simulink model "TST_APP_PlausBrk"  (R2016b)
settings: Solver=FixedStepDiscrete  StartTime=0.0  StopTime=simTime  FixedStep=sampleTime  RelTol=1e-3
values from neighbouring files (symbols this model uses):
  testCase = 1    [initTST_APP_PlausBrk_001.m]    (also in initTST_APP_PlausBrk_002.m = 2; initTST_APP_PlausBrk_003.m = 3; initTST_APP_PlausBrk_004.m = 4; initTST_APP_PlausBrk_005.m = 5)
libraries: simulink x25, UnitTest_Lib x18
(part 1 of 2)
settings Model: Creator=liangyunbo  LastModifiedBy=liangyunbo
settings DebuggingCC: SignalRangeChecking=error

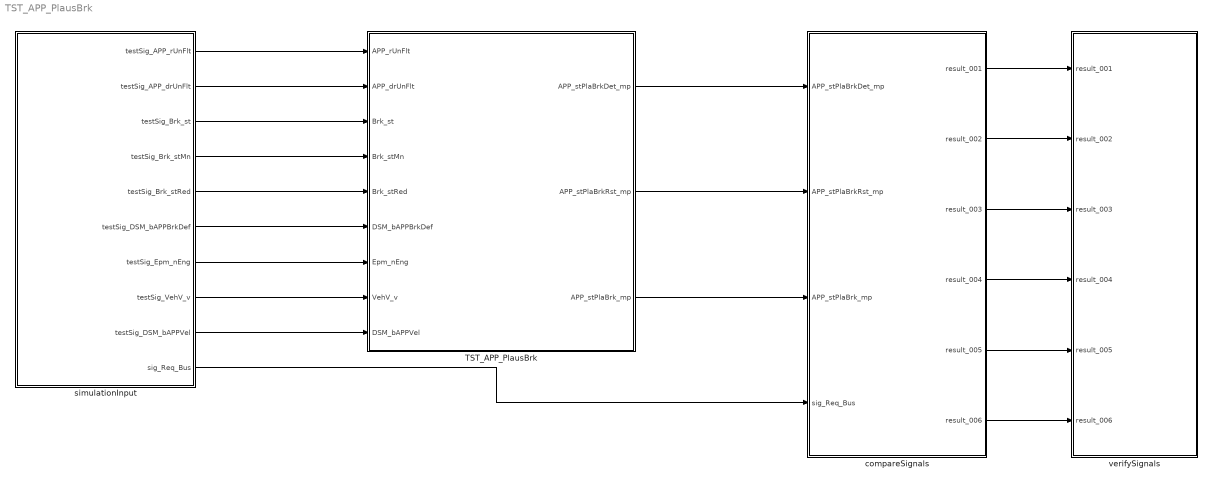
== system TST_APP_PlausBrk ==
  TST_APP_PlausBrk : Subsystem
  compareSignals : Subsystem
  simulationInput : Subsystem
  verifySignals : Subsystem
  wires:
  simulationInput/1(testSig_APP_rUnFlt) -> TST_APP_PlausBrk/1(APP_rUnFlt)
  simulationInput/2(testSig_APP_drUnFlt) -> TST_APP_PlausBrk/2(APP_drUnFlt)
  simulationInput/3(testSig_Brk_st) -> TST_APP_PlausBrk/3(Brk_st)
  simulationInput/4(testSig_Brk_stMn) -> TST_APP_PlausBrk/4(Brk_stMn)
  simulationInput/5(testSig_Brk_stRed) -> TST_APP_PlausBrk/5(Brk_stRed)
  simulationInput/6(testSig_DSM_bAPPBrkDef) -> TST_APP_PlausBrk/6(DSM_bAPPBrkDef)
  simulationInput/7(testSig_Epm_nEng) -> TST_APP_PlausBrk/7(Epm_nEng)
  simulationInput/8(testSig_VehV_v) -> TST_APP_PlausBrk/8(VehV_v)
  simulationInput/9(testSig_DSM_bAPPVel) -> TST_APP_PlausBrk/9(DSM_bAPPVel)
  TST_APP_PlausBrk/1(APP_stPlaBrkDet_mp) -> compareSignals/1(APP_stPlaBrkDet_mp)
  TST_APP_PlausBrk/2(APP_stPlaBrkRst_mp) -> compareSignals/2(APP_stPlaBrkRst_mp)
  TST_APP_PlausBrk/3(APP_stPlaBrk_mp) -> compareSignals/3(APP_stPlaBrk_mp)
  simulationInput/10(sig_Req_Bus) -> compareSignals/4(sig_Req_Bus)
  compareSignals/1(result_001) -> verifySignals/1(result_001)
  compareSignals/2(result_002) -> verifySignals/2(result_002)
  compareSignals/3(result_003) -> verifySignals/3(result_003)
  compareSignals/4(result_004) -> verifySignals/4(result_004)
  compareSignals/5(result_005) -> verifySignals/5(result_005)
  compareSignals/6(result_006) -> verifySignals/6(result_006)

== system TST_APP_PlausBrk/TST_APP_PlausBrk ==
  APP_rUnFlt : Inport
  APP_drUnFlt : Inport  Port=2
  Brk_st : Inport  Port=3
  Brk_stMn : Inport  Port=4
  Brk_stRed : Inport  Port=5
  DSM_bAPPBrkDef : Inport  Port=6
  Epm_nEng : Inport  Port=7
  VehV_v : Inport  Port=8
  DSM_bAPPVel : Inport  Port=9
  APP_PlausBrk : ModelReference  ModelNameDialog=APP_PlausBrk  SimulationMode=Normal  ModelReferenceVersion=1.27  TriggerPortName=function  TriggerPortTriggerType=function-call  TriggerPortStatesWhenEnabling=held
  Function_Call : simulink/Ports & Subsystems/Function-Call Generator  sample_time=sampleTime  numberOfIterations=1
  APP_stPlaBrkDet_mp : Outport
  APP_stPlaBrkRst_mp : Outport  Port=2
  APP_stPlaBrk_mp : Outport  Port=3
  wires:
  Function_Call/1 -> APP_PlausBrk/Trigger
  APP_rUnFlt/1 -> APP_PlausBrk/1
  APP_drUnFlt/1 -> APP_PlausBrk/2
  Brk_st/1 -> APP_PlausBrk/3
  Brk_stMn/1 -> APP_PlausBrk/4
  Brk_stRed/1 -> APP_PlausBrk/5
  DSM_bAPPBrkDef/1 -> APP_PlausBrk/6
  Epm_nEng/1 -> APP_PlausBrk/7
  VehV_v/1 -> APP_PlausBrk/8
  DSM_bAPPVel/1 -> APP_PlausBrk/9
  APP_PlausBrk/1 -> APP_stPlaBrkDet_mp/1
  APP_PlausBrk/2 -> APP_stPlaBrkRst_mp/1
  APP_PlausBrk/3 -> APP_stPlaBrk_mp/1

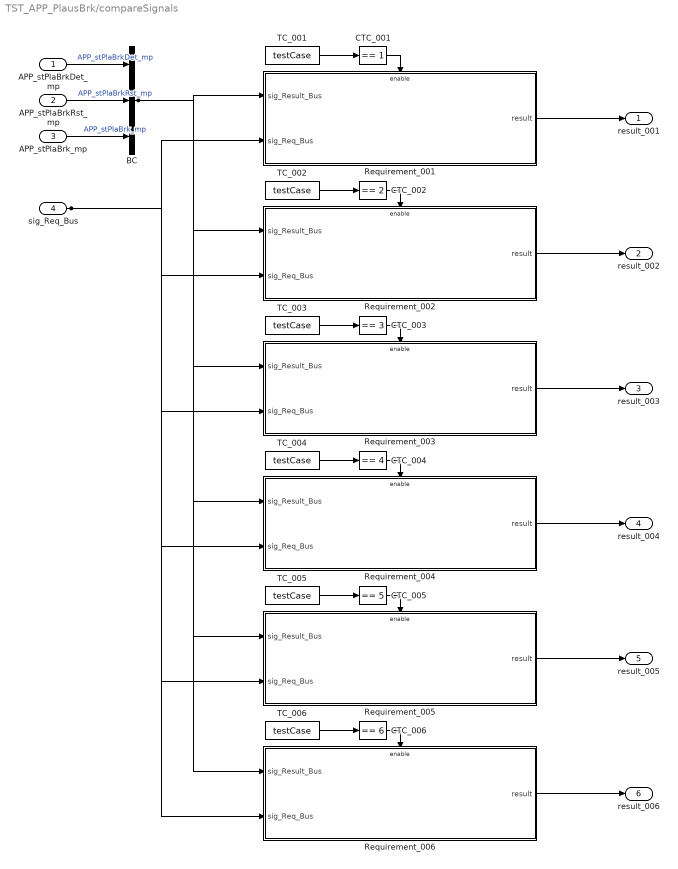
== system TST_APP_PlausBrk/compareSignals ==
  APP_stPlaBrkDet_mp : Inport
  APP_stPlaBrkRst_mp : Inport  Port=2
  APP_stPlaBrk_mp : Inport  Port=3
  sig_Req_Bus : Inport  Port=4
  BC : BusCreator  Inputs=3
  CTC_001 : simulink/Logic and Bit Operations/Compare To Constant  relop===  const=1  OutDataTypeStr=boolean
  CTC_002 : simulink/Logic and Bit Operations/Compare To Constant  relop===  const=2  OutDataTypeStr=boolean
  CTC_003 : simulink/Logic and Bit Operations/Compare To Constant  relop===  const=3  OutDataTypeStr=boolean
  CTC_004 : simulink/Logic and Bit Operations/Compare To Constant  relop===  const=4  OutDataTypeStr=boolean
  CTC_005 : simulink/Logic and Bit Operations/Compare To Constant  relop===  const=5  OutDataTypeStr=boolean
  CTC_006 : simulink/Logic and Bit Operations/Compare To Constant  relop===  const=6  OutDataTypeStr=boolean
  Requirement_001 : Subsystem
  Requirement_002 : Subsystem
  Requirement_003 : Subsystem
  Requirement_004 : Subsystem
  Requirement_005 : Subsystem
  Requirement_006 : Subsystem
  TC_001 : Constant  Value=testCase
  TC_002 : Constant  Value=testCase
  TC_003 : Constant  Value=testCase
  TC_004 : Constant  Value=testCase
  TC_005 : Constant  Value=testCase
  TC_006 : Constant  Value=testCase
  result_001 : Outport
  result_002 : Outport  Port=2
  result_003 : Outport  Port=3
  result_004 : Outport  Port=4
  result_005 : Outport  Port=5
  result_006 : Outport  Port=6
  wires:
  APP_stPlaBrkDet_mp/1 -> BC/1  "APP_stPlaBrkDet_mp"
  APP_stPlaBrkRst_mp/1 -> BC/2  "APP_stPlaBrkRst_mp"
  APP_stPlaBrk_mp/1 -> BC/3  "APP_stPlaBrk_mp"
  TC_001/1 -> CTC_001/1
  CTC_001/1 -> Requirement_001/Enable
  sig_Req_Bus/1 -> Requirement_001/2(sig_Req_Bus), Requirement_002/2(sig_Req_Bus), Requirement_003/2(sig_Req_Bus), Requirement_004/2(sig_Req_Bus), Requirement_005/2(sig_Req_Bus), Requirement_006/2(sig_Req_Bus)
  BC/1 -> Requirement_001/1(sig_Result_Bus), Requirement_002/1(sig_Result_Bus), Requirement_003/1(sig_Result_Bus), Requirement_004/1(sig_Result_Bus), Requirement_005/1(sig_Result_Bus), Requirement_006/1(sig_Result_Bus)
  Requirement_001/1(result) -> result_001/1
  TC_002/1 -> CTC_002/1
  CTC_002/1 -> Requirement_002/Enable
  Requirement_002/1(result) -> result_002/1
  TC_003/1 -> CTC_003/1
  CTC_003/1 -> Requirement_003/Enable
  Requirement_003/1(result) -> result_003/1
  TC_004/1 -> CTC_004/1
  CTC_004/1 -> Requirement_004/Enable
  Requirement_004/1(result) -> result_004/1
  TC_005/1 -> CTC_005/1
  CTC_005/1 -> Requirement_005/Enable
  Requirement_005/1(result) -> result_005/1
  TC_006/1 -> CTC_006/1
  CTC_006/1 -> Requirement_006/Enable
  Requirement_006/1(result) -> result_006/1

== system TST_APP_PlausBrk/simulationInput ==
  BS : BusSelector  OutputSignals=testSig_APP_rUnFlt,testSig_APP_drUnFlt,testSig_Brk_st,testSig_Brk_stMn,testSig_Brk_stRed,testSig_DSM_bAPPBrkDef,testSig_Epm_nEng,testSig_VehV_v,testSig_DSM_bAPPVel
  MPSw : MultiPortSwitch  Inputs=6  SaturateOnIntegerOverflow=on  InputSameDT=on
  TestCase : Constant  Value=testCase
  testSignals_R001 : Subsystem
  testSignals_R002 : Subsystem
  testSignals_R003 : Subsystem
  testSignals_R004 : Subsystem
  testSignals_R005 : Subsystem
  testSignals_R006 : Subsystem
  testSig_APP_rUnFlt : Outport
  testSig_APP_drUnFlt : Outport  Port=2
  testSig_Brk_st : Outport  Port=3
  testSig_Brk_stMn : Outport  Port=4
  testSig_Brk_stRed : Outport  Port=5
  testSig_DSM_bAPPBrkDef : Outport  Port=6
  testSig_Epm_nEng : Outport  Port=7
  testSig_VehV_v : Outport  Port=8
  testSig_DSM_bAPPVel : Outport  Port=9
  sig_Req_Bus : Outport  Port=10
  wires:
  BS/1 -> testSig_APP_rUnFlt/1  "<testSig_APP_rUnFlt>"
  BS/2 -> testSig_APP_drUnFlt/1  "<testSig_APP_drUnFlt>"
  BS/3 -> testSig_Brk_st/1  "<testSig_Brk_st>"
  BS/4 -> testSig_Brk_stMn/1  "<testSig_Brk_stMn>"
  BS/5 -> testSig_Brk_stRed/1  "<testSig_Brk_stRed>"
  BS/6 -> testSig_DSM_bAPPBrkDef/1  "<testSig_DSM_bAPPBrkDef>"
  BS/7 -> testSig_Epm_nEng/1  "<testSig_Epm_nEng>"
  BS/8 -> testSig_VehV_v/1  "<testSig_VehV_v>"
  BS/9 -> testSig_DSM_bAPPVel/1  "<testSig_DSM_bAPPVel>"
  MPSw/1 -> BS/1, sig_Req_Bus/1
  TestCase/1 -> MPSw/1
  testSignals_R001/1(testSignals) -> MPSw/2
  testSignals_R002/1(testSignals) -> MPSw/3
  testSignals_R003/1(testSignals) -> MPSw/4
  testSignals_R004/1(testSignals) -> MPSw/5
  testSignals_R005/1(testSignals) -> MPSw/6
  testSignals_R006/1(testSignals) -> MPSw/7

== system TST_APP_PlausBrk/verifySignals ==
  result_001 : Inport
  result_002 : Inport  Port=2
  result_003 : Inport  Port=3
  result_004 : Inport  Port=4
  result_005 : Inport  Port=5
  result_006 : Inport  Port=6
  Assertion_001 : Assertion  Enabled=off
  Assertion_002 : Assertion  Enabled=off
  Assertion_003 : Assertion  Enabled=off
  Assertion_004 : Assertion  Enabled=off
  Assertion_005 : Assertion  Enabled=off
  Assertion_006 : Assertion  Enabled=off
  wires:
  result_001/1 -> Assertion_001/1
  result_002/1 -> Assertion_002/1
  result_003/1 -> Assertion_003/1
  result_004/1 -> Assertion_004/1
  result_005/1 -> Assertion_005/1
  result_006/1 -> Assertion_006/1

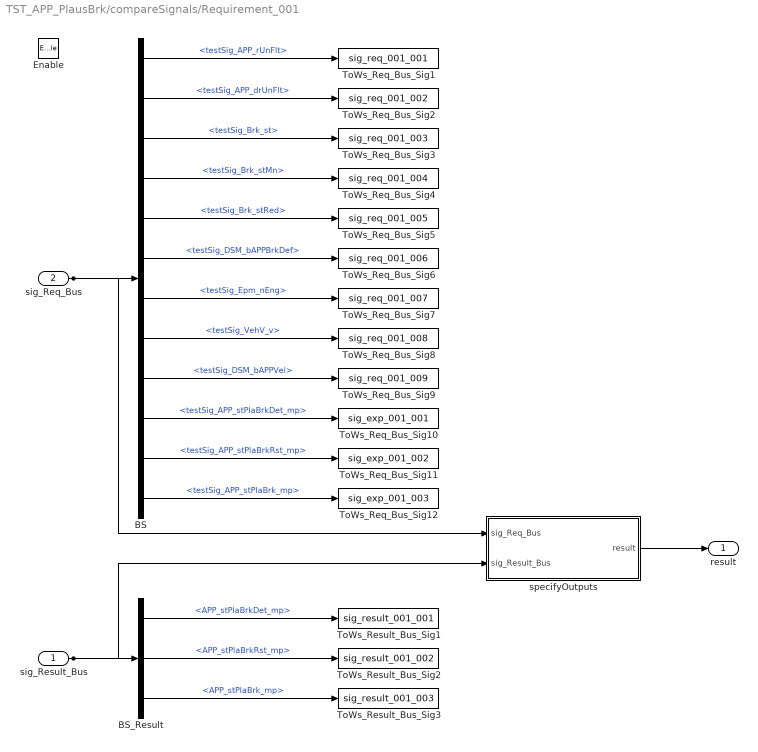
== system TST_APP_PlausBrk/compareSignals/Requirement_001 ==
  sig_Result_Bus : Inport
  sig_Req_Bus : Inport  Port=2
  Enable : EnablePort
  BS : BusSelector  OutputSignals=testSig_APP_rUnFlt,testSig_APP_drUnFlt,testSig_Brk_st,testSig_Brk_stMn,testSig_Brk_stRed,testSig_DSM_bAPPBrkDef,testSig_Epm_nEng,testSig_VehV_v,testSig_DSM_bAPPVel,testSig_APP_stPlaBrkDet_mp,testSig_APP_stPlaBrkRst_mp,testSig_APP_stPlaBrk_mp
  BS_Result : BusSelector  OutputSignals=APP_stPlaBrkDet_mp,APP_stPlaBrkRst_mp,APP_stPlaBrk_mp
  ToWs_Req_Bus_Sig1 : ToWorkspace  VariableName=sig_req_001_001  SaveFormat=Structure With Time
  ToWs_Req_Bus_Sig10 : ToWorkspace  VariableName=sig_exp_001_001  SaveFormat=Structure With Time
  ToWs_Req_Bus_Sig11 : ToWorkspace  VariableName=sig_exp_001_002  SaveFormat=Structure With Time
  ToWs_Req_Bus_Sig12 : ToWorkspace  VariableName=sig_exp_001_003  SaveFormat=Structure With Time
  ToWs_Req_Bus_Sig2 : ToWorkspace  VariableName=sig_req_001_002  SaveFormat=Structure With Time
  ToWs_Req_Bus_Sig3 : ToWorkspace  VariableName=sig_req_001_003  SaveFormat=Structure With Time
  ToWs_Req_Bus_Sig4 : ToWorkspace  VariableName=sig_req_001_004  SaveFormat=Structure With Time
  ToWs_Req_Bus_Sig5 : ToWorkspace  VariableName=sig_req_001_005  SaveFormat=Structure With Time
  ToWs_Req_Bus_Sig6 : ToWorkspace  VariableName=sig_req_001_006  SaveFormat=Structure With Time
  ToWs_Req_Bus_Sig7 : ToWorkspace  VariableName=sig_req_001_007  SaveFormat=Structure With Time
  ToWs_Req_Bus_Sig8 : ToWorkspace  VariableName=sig_req_001_008  SaveFormat=Structure With Time
  ToWs_Req_Bus_Sig9 : ToWorkspace  VariableName=sig_req_001_009  SaveFormat=Structure With Time
  ToWs_Result_Bus_Sig1 : ToWorkspace  VariableName=sig_result_001_001  SaveFormat=Structure With Time
  ToWs_Result_Bus_Sig2 : ToWorkspace  VariableName=sig_result_001_002  SaveFormat=Structure With Time
  ToWs_Result_Bus_Sig3 : ToWorkspace  VariableName=sig_result_001_003  SaveFormat=Structure With Time
  specifyOutputs : Subsystem
  result : Outport
  wires:
  sig_Req_Bus/1 -> BS/1, specifyOutputs/1(sig_Req_Bus)
  BS/1 -> ToWs_Req_Bus_Sig1/1  "<testSig_APP_rUnFlt>"
  BS/2 -> ToWs_Req_Bus_Sig2/1  "<testSig_APP_drUnFlt>"
  BS/3 -> ToWs_Req_Bus_Sig3/1  "<testSig_Brk_st>"
  BS/4 -> ToWs_Req_Bus_Sig4/1  "<testSig_Brk_stMn>"
  BS/5 -> ToWs_Req_Bus_Sig5/1  "<testSig_Brk_stRed>"
  BS/6 -> ToWs_Req_Bus_Sig6/1  "<testSig_DSM_bAPPBrkDef>"
  BS/7 -> ToWs_Req_Bus_Sig7/1  "<testSig_Epm_nEng>"
  BS/8 -> ToWs_Req_Bus_Sig8/1  "<testSig_VehV_v>"
  BS/9 -> ToWs_Req_Bus_Sig9/1  "<testSig_DSM_bAPPVel>"
  BS/10 -> ToWs_Req_Bus_Sig10/1  "<testSig_APP_stPlaBrkDet_mp>"
  BS/11 -> ToWs_Req_Bus_Sig11/1  "<testSig_APP_stPlaBrkRst_mp>"
  BS/12 -> ToWs_Req_Bus_Sig12/1  "<testSig_APP_stPlaBrk_mp>"
  sig_Result_Bus/1 -> BS_Result/1, specifyOutputs/2(sig_Result_Bus)
  BS_Result/1 -> ToWs_Result_Bus_Sig1/1  "<APP_stPlaBrkDet_mp>"
  BS_Result/2 -> ToWs_Result_Bus_Sig2/1  "<APP_stPlaBrkRst_mp>"
  BS_Result/3 -> ToWs_Result_Bus_Sig3/1  "<APP_stPlaBrk_mp>"
  specifyOutputs/1(result) -> result/1

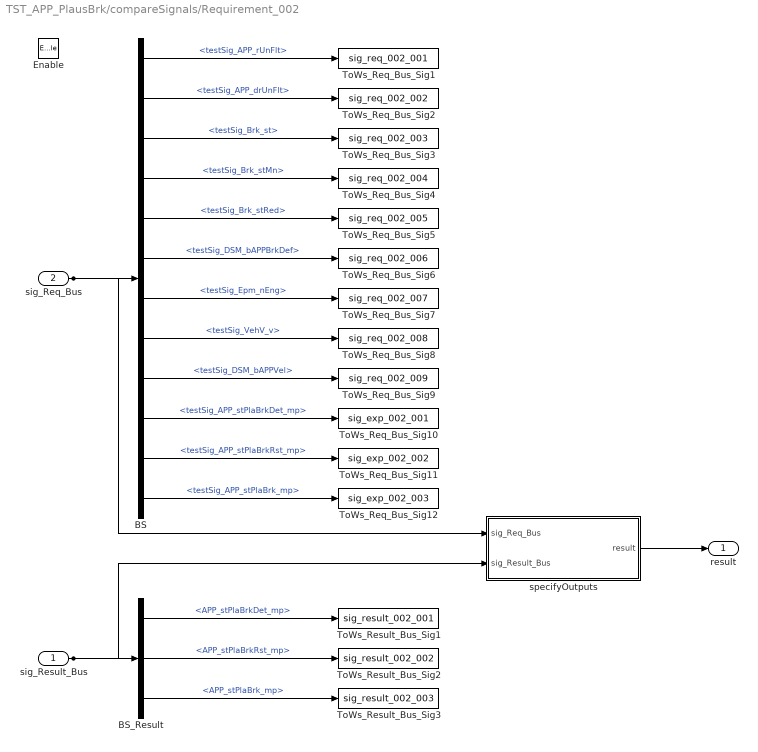
== system TST_APP_PlausBrk/compareSignals/Requirement_002 ==
  sig_Result_Bus : Inport
  sig_Req_Bus : Inport  Port=2
  Enable : EnablePort
  BS : BusSelector  OutputSignals=testSig_APP_rUnFlt,testSig_APP_drUnFlt,testSig_Brk_st,testSig_Brk_stMn,testSig_Brk_stRed,testSig_DSM_bAPPBrkDef,testSig_Epm_nEng,testSig_VehV_v,testSig_DSM_bAPPVel,testSig_APP_stPlaBrkDet_mp,testSig_APP_stPlaBrkRst_mp,testSig_APP_stPlaBrk_mp
  BS_Result : BusSelector  OutputSignals=APP_stPlaBrkDet_mp,APP_stPlaBrkRst_mp,APP_stPlaBrk_mp
  ToWs_Req_Bus_Sig1 : ToWorkspace  VariableName=sig_req_002_001  SaveFormat=Structure With Time
  ToWs_Req_Bus_Sig10 : ToWorkspace  VariableName=sig_exp_002_001  SaveFormat=Structure With Time
  ToWs_Req_Bus_Sig11 : ToWorkspace  VariableName=sig_exp_002_002  SaveFormat=Structure With Time
  ToWs_Req_Bus_Sig12 : ToWorkspace  VariableName=sig_exp_002_003  SaveFormat=Structure With Time
  ToWs_Req_Bus_Sig2 : ToWorkspace  VariableName=sig_req_002_002  SaveFormat=Structure With Time
  ToWs_Req_Bus_Sig3 : ToWorkspace  VariableName=sig_req_002_003  SaveFormat=Structure With Time
  ToWs_Req_Bus_Sig4 : ToWorkspace  VariableName=sig_req_002_004  SaveFormat=Structure With Time
  ToWs_Req_Bus_Sig5 : ToWorkspace  VariableName=sig_req_002_005  SaveFormat=Structure With Time
  ToWs_Req_Bus_Sig6 : ToWorkspace  VariableName=sig_req_002_006  SaveFormat=Structure With Time
  ToWs_Req_Bus_Sig7 : ToWorkspace  VariableName=sig_req_002_007  SaveFormat=Structure With Time
  ToWs_Req_Bus_Sig8 : ToWorkspace  VariableName=sig_req_002_008  SaveFormat=Structure With Time
  ToWs_Req_Bus_Sig9 : ToWorkspace  VariableName=sig_req_002_009  SaveFormat=Structure With Time
  ToWs_Result_Bus_Sig1 : ToWorkspace  VariableName=sig_result_002_001  SaveFormat=Structure With Time
  ToWs_Result_Bus_Sig2 : ToWorkspace  VariableName=sig_result_002_002  SaveFormat=Structure With Time
  ToWs_Result_Bus_Sig3 : ToWorkspace  VariableName=sig_result_002_003  SaveFormat=Structure With Time
  specifyOutputs : Subsystem
  result : Outport
  wires:
  sig_Req_Bus/1 -> BS/1, specifyOutputs/1(sig_Req_Bus)
  BS/1 -> ToWs_Req_Bus_Sig1/1  "<testSig_APP_rUnFlt>"
  BS/2 -> ToWs_Req_Bus_Sig2/1  "<testSig_APP_drUnFlt>"
  BS/3 -> ToWs_Req_Bus_Sig3/1  "<testSig_Brk_st>"
  BS/4 -> ToWs_Req_Bus_Sig4/1  "<testSig_Brk_stMn>"
  BS/5 -> ToWs_Req_Bus_Sig5/1  "<testSig_Brk_stRed>"
  BS/6 -> ToWs_Req_Bus_Sig6/1  "<testSig_DSM_bAPPBrkDef>"
  BS/7 -> ToWs_Req_Bus_Sig7/1  "<testSig_Epm_nEng>"
  BS/8 -> ToWs_Req_Bus_Sig8/1  "<testSig_VehV_v>"
  BS/9 -> ToWs_Req_Bus_Sig9/1  "<testSig_DSM_bAPPVel>"
  BS/10 -> ToWs_Req_Bus_Sig10/1  "<testSig_APP_stPlaBrkDet_mp>"
  BS/11 -> ToWs_Req_Bus_Sig11/1  "<testSig_APP_stPlaBrkRst_mp>"
  BS/12 -> ToWs_Req_Bus_Sig12/1  "<testSig_APP_stPlaBrk_mp>"
  sig_Result_Bus/1 -> BS_Result/1, specifyOutputs/2(sig_Result_Bus)
  BS_Result/1 -> ToWs_Result_Bus_Sig1/1  "<APP_stPlaBrkDet_mp>"
  BS_Result/2 -> ToWs_Result_Bus_Sig2/1  "<APP_stPlaBrkRst_mp>"
  BS_Result/3 -> ToWs_Result_Bus_Sig3/1  "<APP_stPlaBrk_mp>"
  specifyOutputs/1(result) -> result/1

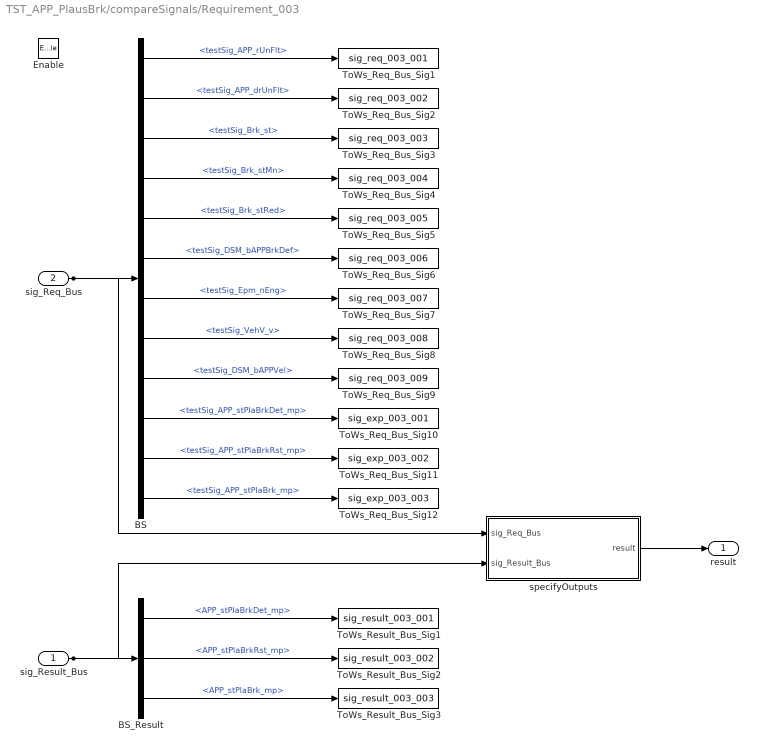
== system TST_APP_PlausBrk/compareSignals/Requirement_003 ==
  sig_Result_Bus : Inport
  sig_Req_Bus : Inport  Port=2
  Enable : EnablePort
  BS : BusSelector  OutputSignals=testSig_APP_rUnFlt,testSig_APP_drUnFlt,testSig_Brk_st,testSig_Brk_stMn,testSig_Brk_stRed,testSig_DSM_bAPPBrkDef,testSig_Epm_nEng,testSig_VehV_v,testSig_DSM_bAPPVel,testSig_APP_stPlaBrkDet_mp,testSig_APP_stPlaBrkRst_mp,testSig_APP_stPlaBrk_mp
  BS_Result : BusSelector  OutputSignals=APP_stPlaBrkDet_mp,APP_stPlaBrkRst_mp,APP_stPlaBrk_mp
  ToWs_Req_Bus_Sig1 : ToWorkspace  VariableName=sig_req_003_001  SaveFormat=Structure With Time
  ToWs_Req_Bus_Sig10 : ToWorkspace  VariableName=sig_exp_003_001  SaveFormat=Structure With Time
  ToWs_Req_Bus_Sig11 : ToWorkspace  VariableName=sig_exp_003_002  SaveFormat=Structure With Time
  ToWs_Req_Bus_Sig12 : ToWorkspace  VariableName=sig_exp_003_003  SaveFormat=Structure With Time
  ToWs_Req_Bus_Sig2 : ToWorkspace  VariableName=sig_req_003_002  SaveFormat=Structure With Time
  ToWs_Req_Bus_Sig3 : ToWorkspace  VariableName=sig_req_003_003  SaveFormat=Structure With Time
  ToWs_Req_Bus_Sig4 : ToWorkspace  VariableName=sig_req_003_004  SaveFormat=Structure With Time
  ToWs_Req_Bus_Sig5 : ToWorkspace  VariableName=sig_req_003_005  SaveFormat=Structure With Time
  ToWs_Req_Bus_Sig6 : ToWorkspace  VariableName=sig_req_003_006  SaveFormat=Structure With Time
  ToWs_Req_Bus_Sig7 : ToWorkspace  VariableName=sig_req_003_007  SaveFormat=Structure With Time
  ToWs_Req_Bus_Sig8 : ToWorkspace  VariableName=sig_req_003_008  SaveFormat=Structure With Time
  ToWs_Req_Bus_Sig9 : ToWorkspace  VariableName=sig_req_003_009  SaveFormat=Structure With Time
  ToWs_Result_Bus_Sig1 : ToWorkspace  VariableName=sig_result_003_001  SaveFormat=Structure With Time
  ToWs_Result_Bus_Sig2 : ToWorkspace  VariableName=sig_result_003_002  SaveFormat=Structure With Time
  ToWs_Result_Bus_Sig3 : ToWorkspace  VariableName=sig_result_003_003  SaveFormat=Structure With Time
  specifyOutputs : Subsystem
  result : Outport
  wires:
  sig_Req_Bus/1 -> BS/1, specifyOutputs/1(sig_Req_Bus)
  BS/1 -> ToWs_Req_Bus_Sig1/1  "<testSig_APP_rUnFlt>"
  BS/2 -> ToWs_Req_Bus_Sig2/1  "<testSig_APP_drUnFlt>"
  BS/3 -> ToWs_Req_Bus_Sig3/1  "<testSig_Brk_st>"
  BS/4 -> ToWs_Req_Bus_Sig4/1  "<testSig_Brk_stMn>"
  BS/5 -> ToWs_Req_Bus_Sig5/1  "<testSig_Brk_stRed>"
  BS/6 -> ToWs_Req_Bus_Sig6/1  "<testSig_DSM_bAPPBrkDef>"
  BS/7 -> ToWs_Req_Bus_Sig7/1  "<testSig_Epm_nEng>"
  BS/8 -> ToWs_Req_Bus_Sig8/1  "<testSig_VehV_v>"
  BS/9 -> ToWs_Req_Bus_Sig9/1  "<testSig_DSM_bAPPVel>"
  BS/10 -> ToWs_Req_Bus_Sig10/1  "<testSig_APP_stPlaBrkDet_mp>"
  BS/11 -> ToWs_Req_Bus_Sig11/1  "<testSig_APP_stPlaBrkRst_mp>"
  BS/12 -> ToWs_Req_Bus_Sig12/1  "<testSig_APP_stPlaBrk_mp>"
  sig_Result_Bus/1 -> BS_Result/1, specifyOutputs/2(sig_Result_Bus)
  BS_Result/1 -> ToWs_Result_Bus_Sig1/1  "<APP_stPlaBrkDet_mp>"
  BS_Result/2 -> ToWs_Result_Bus_Sig2/1  "<APP_stPlaBrkRst_mp>"
  BS_Result/3 -> ToWs_Result_Bus_Sig3/1  "<APP_stPlaBrk_mp>"
  specifyOutputs/1(result) -> result/1

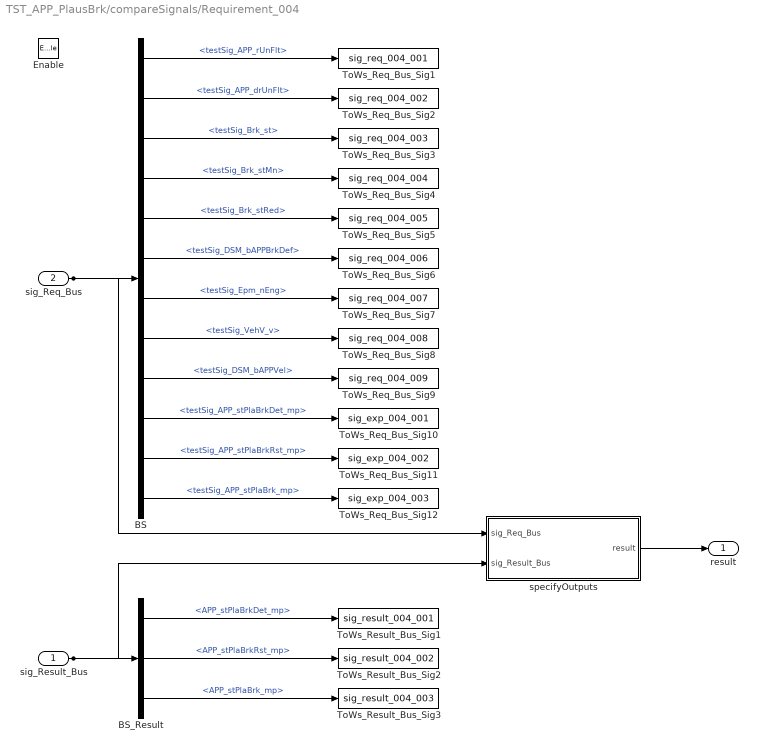
== system TST_APP_PlausBrk/compareSignals/Requirement_004 ==
  sig_Result_Bus : Inport
  sig_Req_Bus : Inport  Port=2
  Enable : EnablePort
  BS : BusSelector  OutputSignals=testSig_APP_rUnFlt,testSig_APP_drUnFlt,testSig_Brk_st,testSig_Brk_stMn,testSig_Brk_stRed,testSig_DSM_bAPPBrkDef,testSig_Epm_nEng,testSig_VehV_v,testSig_DSM_bAPPVel,testSig_APP_stPlaBrkDet_mp,testSig_APP_stPlaBrkRst_mp,testSig_APP_stPlaBrk_mp
  BS_Result : BusSelector  OutputSignals=APP_stPlaBrkDet_mp,APP_stPlaBrkRst_mp,APP_stPlaBrk_mp
  ToWs_Req_Bus_Sig1 : ToWorkspace  VariableName=sig_req_004_001  SaveFormat=Structure With Time
  ToWs_Req_Bus_Sig10 : ToWorkspace  VariableName=sig_exp_004_001  SaveFormat=Structure With Time
  ToWs_Req_Bus_Sig11 : ToWorkspace  VariableName=sig_exp_004_002  SaveFormat=Structure With Time
  ToWs_Req_Bus_Sig12 : ToWorkspace  VariableName=sig_exp_004_003  SaveFormat=Structure With Time
  ToWs_Req_Bus_Sig2 : ToWorkspace  VariableName=sig_req_004_002  SaveFormat=Structure With Time
  ToWs_Req_Bus_Sig3 : ToWorkspace  VariableName=sig_req_004_003  SaveFormat=Structure With Time
  ToWs_Req_Bus_Sig4 : ToWorkspace  VariableName=sig_req_004_004  SaveFormat=Structure With Time
  ToWs_Req_Bus_Sig5 : ToWorkspace  VariableName=sig_req_004_005  SaveFormat=Structure With Time
  ToWs_Req_Bus_Sig6 : ToWorkspace  VariableName=sig_req_004_006  SaveFormat=Structure With Time
  ToWs_Req_Bus_Sig7 : ToWorkspace  VariableName=sig_req_004_007  SaveFormat=Structure With Time
  ToWs_Req_Bus_Sig8 : ToWorkspace  VariableName=sig_req_004_008  SaveFormat=Structure With Time
  ToWs_Req_Bus_Sig9 : ToWorkspace  VariableName=sig_req_004_009  SaveFormat=Structure With Time
  ToWs_Result_Bus_Sig1 : ToWorkspace  VariableName=sig_result_004_001  SaveFormat=Structure With Time
  ToWs_Result_Bus_Sig2 : ToWorkspace  VariableName=sig_result_004_002  SaveFormat=Structure With Time
  ToWs_Result_Bus_Sig3 : ToWorkspace  VariableName=sig_result_004_003  SaveFormat=Structure With Time
  specifyOutputs : Subsystem
  result : Outport
  wires:
  sig_Req_Bus/1 -> BS/1, specifyOutputs/1(sig_Req_Bus)
  BS/1 -> ToWs_Req_Bus_Sig1/1  "<testSig_APP_rUnFlt>"
  BS/2 -> ToWs_Req_Bus_Sig2/1  "<testSig_APP_drUnFlt>"
  BS/3 -> ToWs_Req_Bus_Sig3/1  "<testSig_Brk_st>"
  BS/4 -> ToWs_Req_Bus_Sig4/1  "<testSig_Brk_stMn>"
  BS/5 -> ToWs_Req_Bus_Sig5/1  "<testSig_Brk_stRed>"
  BS/6 -> ToWs_Req_Bus_Sig6/1  "<testSig_DSM_bAPPBrkDef>"
  BS/7 -> ToWs_Req_Bus_Sig7/1  "<testSig_Epm_nEng>"
  BS/8 -> ToWs_Req_Bus_Sig8/1  "<testSig_VehV_v>"
  BS/9 -> ToWs_Req_Bus_Sig9/1  "<testSig_DSM_bAPPVel>"
  BS/10 -> ToWs_Req_Bus_Sig10/1  "<testSig_APP_stPlaBrkDet_mp>"
  BS/11 -> ToWs_Req_Bus_Sig11/1  "<testSig_APP_stPlaBrkRst_mp>"
  BS/12 -> ToWs_Req_Bus_Sig12/1  "<testSig_APP_stPlaBrk_mp>"
  sig_Result_Bus/1 -> BS_Result/1, specifyOutputs/2(sig_Result_Bus)
  BS_Result/1 -> ToWs_Result_Bus_Sig1/1  "<APP_stPlaBrkDet_mp>"
  BS_Result/2 -> ToWs_Result_Bus_Sig2/1  "<APP_stPlaBrkRst_mp>"
  BS_Result/3 -> ToWs_Result_Bus_Sig3/1  "<APP_stPlaBrk_mp>"
  specifyOutputs/1(result) -> result/1

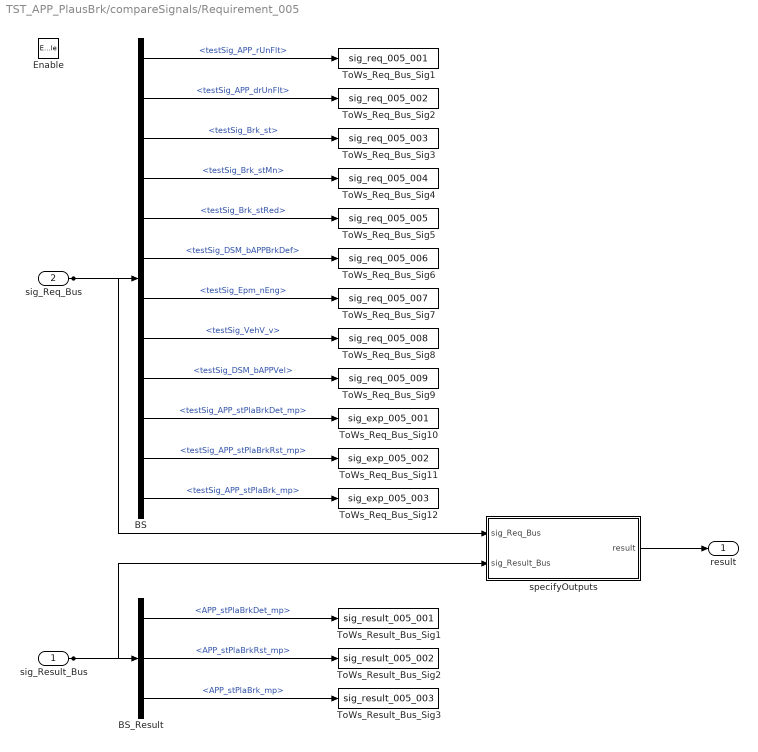
== system TST_APP_PlausBrk/compareSignals/Requirement_005 ==
  sig_Result_Bus : Inport
  sig_Req_Bus : Inport  Port=2
  Enable : EnablePort
  BS : BusSelector  OutputSignals=testSig_APP_rUnFlt,testSig_APP_drUnFlt,testSig_Brk_st,testSig_Brk_stMn,testSig_Brk_stRed,testSig_DSM_bAPPBrkDef,testSig_Epm_nEng,testSig_VehV_v,testSig_DSM_bAPPVel,testSig_APP_stPlaBrkDet_mp,testSig_APP_stPlaBrkRst_mp,testSig_APP_stPlaBrk_mp
  BS_Result : BusSelector  OutputSignals=APP_stPlaBrkDet_mp,APP_stPlaBrkRst_mp,APP_stPlaBrk_mp
  ToWs_Req_Bus_Sig1 : ToWorkspace  VariableName=sig_req_005_001  SaveFormat=Structure With Time
  ToWs_Req_Bus_Sig10 : ToWorkspace  VariableName=sig_exp_005_001  SaveFormat=Structure With Time
  ToWs_Req_Bus_Sig11 : ToWorkspace  VariableName=sig_exp_005_002  SaveFormat=Structure With Time
  ToWs_Req_Bus_Sig12 : ToWorkspace  VariableName=sig_exp_005_003  SaveFormat=Structure With Time
  ToWs_Req_Bus_Sig2 : ToWorkspace  VariableName=sig_req_005_002  SaveFormat=Structure With Time
  ToWs_Req_Bus_Sig3 : ToWorkspace  VariableName=sig_req_005_003  SaveFormat=Structure With Time
  ToWs_Req_Bus_Sig4 : ToWorkspace  VariableName=sig_req_005_004  SaveFormat=Structure With Time
  ToWs_Req_Bus_Sig5 : ToWorkspace  VariableName=sig_req_005_005  SaveFormat=Structure With Time
  ToWs_Req_Bus_Sig6 : ToWorkspace  VariableName=sig_req_005_006  SaveFormat=Structure With Time
  ToWs_Req_Bus_Sig7 : ToWorkspace  VariableName=sig_req_005_007  SaveFormat=Structure With Time
  ToWs_Req_Bus_Sig8 : ToWorkspace  VariableName=sig_req_005_008  SaveFormat=Structure With Time
  ToWs_Req_Bus_Sig9 : ToWorkspace  VariableName=sig_req_005_009  SaveFormat=Structure With Time
  ToWs_Result_Bus_Sig1 : ToWorkspace  VariableName=sig_result_005_001  SaveFormat=Structure With Time
  ToWs_Result_Bus_Sig2 : ToWorkspace  VariableName=sig_result_005_002  SaveFormat=Structure With Time
  ToWs_Result_Bus_Sig3 : ToWorkspace  VariableName=sig_result_005_003  SaveFormat=Structure With Time
  specifyOutputs : Subsystem
  result : Outport
  wires:
  sig_Req_Bus/1 -> BS/1, specifyOutputs/1(sig_Req_Bus)
  BS/1 -> ToWs_Req_Bus_Sig1/1  "<testSig_APP_rUnFlt>"
  BS/2 -> ToWs_Req_Bus_Sig2/1  "<testSig_APP_drUnFlt>"
  BS/3 -> ToWs_Req_Bus_Sig3/1  "<testSig_Brk_st>"
  BS/4 -> ToWs_Req_Bus_Sig4/1  "<testSig_Brk_stMn>"
  BS/5 -> ToWs_Req_Bus_Sig5/1  "<testSig_Brk_stRed>"
  BS/6 -> ToWs_Req_Bus_Sig6/1  "<testSig_DSM_bAPPBrkDef>"
  BS/7 -> ToWs_Req_Bus_Sig7/1  "<testSig_Epm_nEng>"
  BS/8 -> ToWs_Req_Bus_Sig8/1  "<testSig_VehV_v>"
  BS/9 -> ToWs_Req_Bus_Sig9/1  "<testSig_DSM_bAPPVel>"
  BS/10 -> ToWs_Req_Bus_Sig10/1  "<testSig_APP_stPlaBrkDet_mp>"
  BS/11 -> ToWs_Req_Bus_Sig11/1  "<testSig_APP_stPlaBrkRst_mp>"
  BS/12 -> ToWs_Req_Bus_Sig12/1  "<testSig_APP_stPlaBrk_mp>"
  sig_Result_Bus/1 -> BS_Result/1, specifyOutputs/2(sig_Result_Bus)
  BS_Result/1 -> ToWs_Result_Bus_Sig1/1  "<APP_stPlaBrkDet_mp>"
  BS_Result/2 -> ToWs_Result_Bus_Sig2/1  "<APP_stPlaBrkRst_mp>"
  BS_Result/3 -> ToWs_Result_Bus_Sig3/1  "<APP_stPlaBrk_mp>"
  specifyOutputs/1(result) -> result/1

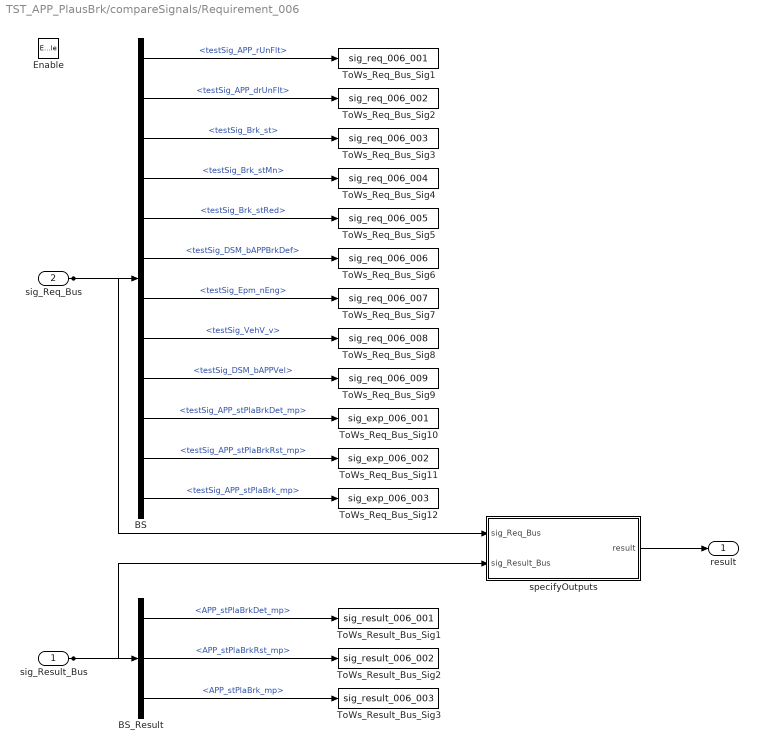
== system TST_APP_PlausBrk/compareSignals/Requirement_006 ==
  sig_Result_Bus : Inport
  sig_Req_Bus : Inport  Port=2
  Enable : EnablePort
  BS : BusSelector  OutputSignals=testSig_APP_rUnFlt,testSig_APP_drUnFlt,testSig_Brk_st,testSig_Brk_stMn,testSig_Brk_stRed,testSig_DSM_bAPPBrkDef,testSig_Epm_nEng,testSig_VehV_v,testSig_DSM_bAPPVel,testSig_APP_stPlaBrkDet_mp,testSig_APP_stPlaBrkRst_mp,testSig_APP_stPlaBrk_mp
  BS_Result : BusSelector  OutputSignals=APP_stPlaBrkDet_mp,APP_stPlaBrkRst_mp,APP_stPlaBrk_mp
  ToWs_Req_Bus_Sig1 : ToWorkspace  VariableName=sig_req_006_001  SaveFormat=Structure With Time
  ToWs_Req_Bus_Sig10 : ToWorkspace  VariableName=sig_exp_006_001  SaveFormat=Structure With Time
  ToWs_Req_Bus_Sig11 : ToWorkspace  VariableName=sig_exp_006_002  SaveFormat=Structure With Time
  ToWs_Req_Bus_Sig12 : ToWorkspace  VariableName=sig_exp_006_003  SaveFormat=Structure With Time
  ToWs_Req_Bus_Sig2 : ToWorkspace  VariableName=sig_req_006_002  SaveFormat=Structure With Time
  ToWs_Req_Bus_Sig3 : ToWorkspace  VariableName=sig_req_006_003  SaveFormat=Structure With Time
  ToWs_Req_Bus_Sig4 : ToWorkspace  VariableName=sig_req_006_004  SaveFormat=Structure With Time
  ToWs_Req_Bus_Sig5 : ToWorkspace  VariableName=sig_req_006_005  SaveFormat=Structure With Time
  ToWs_Req_Bus_Sig6 : ToWorkspace  VariableName=sig_req_006_006  SaveFormat=Structure With Time
  ToWs_Req_Bus_Sig7 : ToWorkspace  VariableName=sig_req_006_007  SaveFormat=Structure With Time
  ToWs_Req_Bus_Sig8 : ToWorkspace  VariableName=sig_req_006_008  SaveFormat=Structure With Time
  ToWs_Req_Bus_Sig9 : ToWorkspace  VariableName=sig_req_006_009  SaveFormat=Structure With Time
  ToWs_Result_Bus_Sig1 : ToWorkspace  VariableName=sig_result_006_001  SaveFormat=Structure With Time
  ToWs_Result_Bus_Sig2 : ToWorkspace  VariableName=sig_result_006_002  SaveFormat=Structure With Time
  ToWs_Result_Bus_Sig3 : ToWorkspace  VariableName=sig_result_006_003  SaveFormat=Structure With Time
  specifyOutputs : Subsystem
  result : Outport
  wires:
  sig_Req_Bus/1 -> BS/1, specifyOutputs/1(sig_Req_Bus)
  BS/1 -> ToWs_Req_Bus_Sig1/1  "<testSig_APP_rUnFlt>"
  BS/2 -> ToWs_Req_Bus_Sig2/1  "<testSig_APP_drUnFlt>"
  BS/3 -> ToWs_Req_Bus_Sig3/1  "<testSig_Brk_st>"
  BS/4 -> ToWs_Req_Bus_Sig4/1  "<testSig_Brk_stMn>"
  BS/5 -> ToWs_Req_Bus_Sig5/1  "<testSig_Brk_stRed>"
  BS/6 -> ToWs_Req_Bus_Sig6/1  "<testSig_DSM_bAPPBrkDef>"
  BS/7 -> ToWs_Req_Bus_Sig7/1  "<testSig_Epm_nEng>"
  BS/8 -> ToWs_Req_Bus_Sig8/1  "<testSig_VehV_v>"
  BS/9 -> ToWs_Req_Bus_Sig9/1  "<testSig_DSM_bAPPVel>"
  BS/10 -> ToWs_Req_Bus_Sig10/1  "<testSig_APP_stPlaBrkDet_mp>"
  BS/11 -> ToWs_Req_Bus_Sig11/1  "<testSig_APP_stPlaBrkRst_mp>"
  BS/12 -> ToWs_Req_Bus_Sig12/1  "<testSig_APP_stPlaBrk_mp>"
  sig_Result_Bus/1 -> BS_Result/1, specifyOutputs/2(sig_Result_Bus)
  BS_Result/1 -> ToWs_Result_Bus_Sig1/1  "<APP_stPlaBrkDet_mp>"
  BS_Result/2 -> ToWs_Result_Bus_Sig2/1  "<APP_stPlaBrkRst_mp>"
  BS_Result/3 -> ToWs_Result_Bus_Sig3/1  "<APP_stPlaBrk_mp>"
  specifyOutputs/1(result) -> result/1

== system TST_APP_PlausBrk/simulationInput/testSignals_R001 ==
  BC : BusCreator  Inputs=12
  spec_APP_drUnFlt : FromWorkspace  VariableName=testSig_APP_drUnFlt  Interpolate=off  OutputAfterFinalValue=Holding final value
  spec_APP_rUnFlt : FromWorkspace  VariableName=testSig_APP_rUnFlt  Interpolate=off  OutputAfterFinalValue=Holding final value
  spec_APP_stPlaBrkDet_mp : FromWorkspace  VariableName=testSig_APP_stPlaBrkDet_mp  Interpolate=off  OutputAfterFinalValue=Holding final value
  spec_APP_stPlaBrkRst_mp : FromWorkspace  VariableName=testSig_APP_stPlaBrkRst_mp  Interpolate=off  OutputAfterFinalValue=Holding final value
  spec_APP_stPlaBrk_mp : FromWorkspace  VariableName=testSig_APP_stPlaBrk_mp  Interpolate=off  OutputAfterFinalValue=Holding final value
  spec_Brk_st : FromWorkspace  VariableName=testSig_Brk_st  Interpolate=off  OutputAfterFinalValue=Holding final value
  spec_Brk_stMn : FromWorkspace  VariableName=testSig_Brk_stMn  Interpolate=off  OutputAfterFinalValue=Holding final value
  spec_Brk_stRed : FromWorkspace  VariableName=testSig_Brk_stRed  Interpolate=off  OutputAfterFinalValue=Holding final value
  spec_DSM_bAPPBrkDef : FromWorkspace  VariableName=testSig_DSM_bAPPBrkDef  Interpolate=off  OutputAfterFinalValue=Holding final value
  spec_DSM_bAPPVel : FromWorkspace  VariableName=testSig_DSM_bAPPVel  Interpolate=off  OutputAfterFinalValue=Holding final value
  spec_Epm_nEng : FromWorkspace  VariableName=testSig_Epm_nEng  Interpolate=off  OutputAfterFinalValue=Holding final value
  spec_VehV_v : FromWorkspace  VariableName=testSig_VehV_v  Interpolate=off  OutputAfterFinalValue=Holding final value
  testSignals : Outport
  wires:
  BC/1 -> testSignals/1
  spec_APP_rUnFlt/1 -> BC/1  "testSig_APP_rUnFlt"
  spec_APP_drUnFlt/1 -> BC/2  "testSig_APP_drUnFlt"
  spec_Brk_st/1 -> BC/3  "testSig_Brk_st"
  spec_Brk_stMn/1 -> BC/4  "testSig_Brk_stMn"
  spec_Brk_stRed/1 -> BC/5  "testSig_Brk_stRed"
  spec_DSM_bAPPBrkDef/1 -> BC/6  "testSig_DSM_bAPPBrkDef"
  spec_Epm_nEng/1 -> BC/7  "testSig_Epm_nEng"
  spec_VehV_v/1 -> BC/8  "testSig_VehV_v"
  spec_DSM_bAPPVel/1 -> BC/9  "testSig_DSM_bAPPVel"
  spec_APP_stPlaBrkDet_mp/1 -> BC/10  "testSig_APP_stPlaBrkDet_mp"
  spec_APP_stPlaBrkRst_mp/1 -> BC/11  "testSig_APP_stPlaBrkRst_mp"
  spec_APP_stPlaBrk_mp/1 -> BC/12  "testSig_APP_stPlaBrk_mp"

== system TST_APP_PlausBrk/simulationInput/testSignals_R002 ==
  BC : BusCreator  Inputs=12
  spec_APP_drUnFlt : FromWorkspace  VariableName=testSig_APP_drUnFlt  Interpolate=off  OutputAfterFinalValue=Holding final value
  spec_APP_rUnFlt : FromWorkspace  VariableName=testSig_APP_rUnFlt  Interpolate=off  OutputAfterFinalValue=Holding final value
  spec_APP_stPlaBrkDet_mp : FromWorkspace  VariableName=testSig_APP_stPlaBrkDet_mp  Interpolate=off  OutputAfterFinalValue=Holding final value
  spec_APP_stPlaBrkRst_mp : FromWorkspace  VariableName=testSig_APP_stPlaBrkRst_mp  Interpolate=off  OutputAfterFinalValue=Holding final value
  spec_APP_stPlaBrk_mp : FromWorkspace  VariableName=testSig_APP_stPlaBrk_mp  Interpolate=off  OutputAfterFinalValue=Holding final value
  spec_Brk_st : FromWorkspace  VariableName=testSig_Brk_st  Interpolate=off  OutputAfterFinalValue=Holding final value
  spec_Brk_stMn : FromWorkspace  VariableName=testSig_Brk_stMn  Interpolate=off  OutputAfterFinalValue=Holding final value
  spec_Brk_stRed : FromWorkspace  VariableName=testSig_Brk_stRed  Interpolate=off  OutputAfterFinalValue=Holding final value
  spec_DSM_bAPPBrkDef : FromWorkspace  VariableName=testSig_DSM_bAPPBrkDef  Interpolate=off  OutputAfterFinalValue=Holding final value
  spec_DSM_bAPPVel : FromWorkspace  VariableName=testSig_DSM_bAPPVel  Interpolate=off  OutputAfterFinalValue=Holding final value
  spec_Epm_nEng : FromWorkspace  VariableName=testSig_Epm_nEng  Interpolate=off  OutputAfterFinalValue=Holding final value
  spec_VehV_v : FromWorkspace  VariableName=testSig_VehV_v  Interpolate=off  OutputAfterFinalValue=Holding final value
  testSignals : Outport
  wires:
  BC/1 -> testSignals/1
  spec_APP_rUnFlt/1 -> BC/1  "testSig_APP_rUnFlt"
  spec_APP_drUnFlt/1 -> BC/2  "testSig_APP_drUnFlt"
  spec_Brk_st/1 -> BC/3  "testSig_Brk_st"
  spec_Brk_stMn/1 -> BC/4  "testSig_Brk_stMn"
  spec_Brk_stRed/1 -> BC/5  "testSig_Brk_stRed"
  spec_DSM_bAPPBrkDef/1 -> BC/6  "testSig_DSM_bAPPBrkDef"
  spec_Epm_nEng/1 -> BC/7  "testSig_Epm_nEng"
  spec_VehV_v/1 -> BC/8  "testSig_VehV_v"
  spec_DSM_bAPPVel/1 -> BC/9  "testSig_DSM_bAPPVel"
  spec_APP_stPlaBrkDet_mp/1 -> BC/10  "testSig_APP_stPlaBrkDet_mp"
  spec_APP_stPlaBrkRst_mp/1 -> BC/11  "testSig_APP_stPlaBrkRst_mp"
  spec_APP_stPlaBrk_mp/1 -> BC/12  "testSig_APP_stPlaBrk_mp"

== system TST_APP_PlausBrk/simulationInput/testSignals_R003 ==
  BC : BusCreator  Inputs=12
  spec_APP_drUnFlt : FromWorkspace  VariableName=testSig_APP_drUnFlt  Interpolate=off  OutputAfterFinalValue=Holding final value
  spec_APP_rUnFlt : FromWorkspace  VariableName=testSig_APP_rUnFlt  Interpolate=off  OutputAfterFinalValue=Holding final value
  spec_APP_stPlaBrkDet_mp : FromWorkspace  VariableName=testSig_APP_stPlaBrkDet_mp  Interpolate=off  OutputAfterFinalValue=Holding final value
  spec_APP_stPlaBrkRst_mp : FromWorkspace  VariableName=testSig_APP_stPlaBrkRst_mp  Interpolate=off  OutputAfterFinalValue=Holding final value
  spec_APP_stPlaBrk_mp : FromWorkspace  VariableName=testSig_APP_stPlaBrk_mp  Interpolate=off  OutputAfterFinalValue=Holding final value
  spec_Brk_st : FromWorkspace  VariableName=testSig_Brk_st  Interpolate=off  OutputAfterFinalValue=Holding final value
  spec_Brk_stMn : FromWorkspace  VariableName=testSig_Brk_stMn  Interpolate=off  OutputAfterFinalValue=Holding final value
  spec_Brk_stRed : FromWorkspace  VariableName=testSig_Brk_stRed  Interpolate=off  OutputAfterFinalValue=Holding final value
  spec_DSM_bAPPBrkDef : FromWorkspace  VariableName=testSig_DSM_bAPPBrkDef  Interpolate=off  OutputAfterFinalValue=Holding final value
  spec_DSM_bAPPVel : FromWorkspace  VariableName=testSig_DSM_bAPPVel  Interpolate=off  OutputAfterFinalValue=Holding final value
  spec_Epm_nEng : FromWorkspace  VariableName=testSig_Epm_nEng  Interpolate=off  OutputAfterFinalValue=Holding final value
  spec_VehV_v : FromWorkspace  VariableName=testSig_VehV_v  Interpolate=off  OutputAfterFinalValue=Holding final value
  testSignals : Outport
  wires:
  BC/1 -> testSignals/1
  spec_APP_rUnFlt/1 -> BC/1  "testSig_APP_rUnFlt"
  spec_APP_drUnFlt/1 -> BC/2  "testSig_APP_drUnFlt"
  spec_Brk_st/1 -> BC/3  "testSig_Brk_st"
  spec_Brk_stMn/1 -> BC/4  "testSig_Brk_stMn"
  spec_Brk_stRed/1 -> BC/5  "testSig_Brk_stRed"
  spec_DSM_bAPPBrkDef/1 -> BC/6  "testSig_DSM_bAPPBrkDef"
  spec_Epm_nEng/1 -> BC/7  "testSig_Epm_nEng"
  spec_VehV_v/1 -> BC/8  "testSig_VehV_v"
  spec_DSM_bAPPVel/1 -> BC/9  "testSig_DSM_bAPPVel"
  spec_APP_stPlaBrkDet_mp/1 -> BC/10  "testSig_APP_stPlaBrkDet_mp"
  spec_APP_stPlaBrkRst_mp/1 -> BC/11  "testSig_APP_stPlaBrkRst_mp"
  spec_APP_stPlaBrk_mp/1 -> BC/12  "testSig_APP_stPlaBrk_mp"

== system TST_APP_PlausBrk/simulationInput/testSignals_R004 ==
  BC : BusCreator  Inputs=12
  spec_APP_drUnFlt : FromWorkspace  VariableName=testSig_APP_drUnFlt  Interpolate=off  OutputAfterFinalValue=Holding final value
  spec_APP_rUnFlt : FromWorkspace  VariableName=testSig_APP_rUnFlt  Interpolate=off  OutputAfterFinalValue=Holding final value
  spec_APP_stPlaBrkDet_mp : FromWorkspace  VariableName=testSig_APP_stPlaBrkDet_mp  Interpolate=off  OutputAfterFinalValue=Holding final value
  spec_APP_stPlaBrkRst_mp : FromWorkspace  VariableName=testSig_APP_stPlaBrkRst_mp  Interpolate=off  OutputAfterFinalValue=Holding final value
  spec_APP_stPlaBrk_mp : FromWorkspace  VariableName=testSig_APP_stPlaBrk_mp  Interpolate=off  OutputAfterFinalValue=Holding final value
  spec_Brk_st : FromWorkspace  VariableName=testSig_Brk_st  Interpolate=off  OutputAfterFinalValue=Holding final value
  spec_Brk_stMn : FromWorkspace  VariableName=testSig_Brk_stMn  Interpolate=off  OutputAfterFinalValue=Holding final value
  spec_Brk_stRed : FromWorkspace  VariableName=testSig_Brk_stRed  Interpolate=off  OutputAfterFinalValue=Holding final value
  spec_DSM_bAPPBrkDef : FromWorkspace  VariableName=testSig_DSM_bAPPBrkDef  Interpolate=off  OutputAfterFinalValue=Holding final value
  spec_DSM_bAPPVel : FromWorkspace  VariableName=testSig_DSM_bAPPVel  Interpolate=off  OutputAfterFinalValue=Holding final value
  spec_Epm_nEng : FromWorkspace  VariableName=testSig_Epm_nEng  Interpolate=off  OutputAfterFinalValue=Holding final value
  spec_VehV_v : FromWorkspace  VariableName=testSig_VehV_v  Interpolate=off  OutputAfterFinalValue=Holding final value
  testSignals : Outport
  wires:
  BC/1 -> testSignals/1
  spec_APP_rUnFlt/1 -> BC/1  "testSig_APP_rUnFlt"
  spec_APP_drUnFlt/1 -> BC/2  "testSig_APP_drUnFlt"
  spec_Brk_st/1 -> BC/3  "testSig_Brk_st"
  spec_Brk_stMn/1 -> BC/4  "testSig_Brk_stMn"
  spec_Brk_stRed/1 -> BC/5  "testSig_Brk_stRed"
  spec_DSM_bAPPBrkDef/1 -> BC/6  "testSig_DSM_bAPPBrkDef"
  spec_Epm_nEng/1 -> BC/7  "testSig_Epm_nEng"
  spec_VehV_v/1 -> BC/8  "testSig_VehV_v"
  spec_DSM_bAPPVel/1 -> BC/9  "testSig_DSM_bAPPVel"
  spec_APP_stPlaBrkDet_mp/1 -> BC/10  "testSig_APP_stPlaBrkDet_mp"
  spec_APP_stPlaBrkRst_mp/1 -> BC/11  "testSig_APP_stPlaBrkRst_mp"
  spec_APP_stPlaBrk_mp/1 -> BC/12  "testSig_APP_stPlaBrk_mp"

== system TST_APP_PlausBrk/simulationInput/testSignals_R005 ==
  BC : BusCreator  Inputs=12
  spec_APP_drUnFlt : FromWorkspace  VariableName=testSig_APP_drUnFlt  Interpolate=off  OutputAfterFinalValue=Holding final value
  spec_APP_rUnFlt : FromWorkspace  VariableName=testSig_APP_rUnFlt  Interpolate=off  OutputAfterFinalValue=Holding final value
  spec_APP_stPlaBrkDet_mp : FromWorkspace  VariableName=testSig_APP_stPlaBrkDet_mp  Interpolate=off  OutputAfterFinalValue=Holding final value
  spec_APP_stPlaBrkRst_mp : FromWorkspace  VariableName=testSig_APP_stPlaBrkRst_mp  Interpolate=off  OutputAfterFinalValue=Holding final value
  spec_APP_stPlaBrk_mp : FromWorkspace  VariableName=testSig_APP_stPlaBrk_mp  Interpolate=off  OutputAfterFinalValue=Holding final value
  spec_Brk_st : FromWorkspace  VariableName=testSig_Brk_st  Interpolate=off  OutputAfterFinalValue=Holding final value
  spec_Brk_stMn : FromWorkspace  VariableName=testSig_Brk_stMn  Interpolate=off  OutputAfterFinalValue=Holding final value
  spec_Brk_stRed : FromWorkspace  VariableName=testSig_Brk_stRed  Interpolate=off  OutputAfterFinalValue=Holding final value
  spec_DSM_bAPPBrkDef : FromWorkspace  VariableName=testSig_DSM_bAPPBrkDef  Interpolate=off  OutputAfterFinalValue=Holding final value
  spec_DSM_bAPPVel : FromWorkspace  VariableName=testSig_DSM_bAPPVel  Interpolate=off  OutputAfterFinalValue=Holding final value
  spec_Epm_nEng : FromWorkspace  VariableName=testSig_Epm_nEng  Interpolate=off  OutputAfterFinalValue=Holding final value
  spec_VehV_v : FromWorkspace  VariableName=testSig_VehV_v  Interpolate=off  OutputAfterFinalValue=Holding final value
  testSignals : Outport
  wires:
  BC/1 -> testSignals/1
  spec_APP_rUnFlt/1 -> BC/1  "testSig_APP_rUnFlt"
  spec_APP_drUnFlt/1 -> BC/2  "testSig_APP_drUnFlt"
  spec_Brk_st/1 -> BC/3  "testSig_Brk_st"
  spec_Brk_stMn/1 -> BC/4  "testSig_Brk_stMn"
  spec_Brk_stRed/1 -> BC/5  "testSig_Brk_stRed"
  spec_DSM_bAPPBrkDef/1 -> BC/6  "testSig_DSM_bAPPBrkDef"
  spec_Epm_nEng/1 -> BC/7  "testSig_Epm_nEng"
  spec_VehV_v/1 -> BC/8  "testSig_VehV_v"
  spec_DSM_bAPPVel/1 -> BC/9  "testSig_DSM_bAPPVel"
  spec_APP_stPlaBrkDet_mp/1 -> BC/10  "testSig_APP_stPlaBrkDet_mp"
  spec_APP_stPlaBrkRst_mp/1 -> BC/11  "testSig_APP_stPlaBrkRst_mp"
  spec_APP_stPlaBrk_mp/1 -> BC/12  "testSig_APP_stPlaBrk_mp"

== system TST_APP_PlausBrk/simulationInput/testSignals_R006 ==
  BC : BusCreator  Inputs=12
  spec_APP_drUnFlt : FromWorkspace  VariableName=testSig_APP_drUnFlt  Interpolate=off  OutputAfterFinalValue=Holding final value
  spec_APP_rUnFlt : FromWorkspace  VariableName=testSig_APP_rUnFlt  Interpolate=off  OutputAfterFinalValue=Holding final value
  spec_APP_stPlaBrkDet_mp : FromWorkspace  VariableName=testSig_APP_stPlaBrkDet_mp  Interpolate=off  OutputAfterFinalValue=Holding final value
  spec_APP_stPlaBrkRst_mp : FromWorkspace  VariableName=testSig_APP_stPlaBrkRst_mp  Interpolate=off  OutputAfterFinalValue=Holding final value
  spec_APP_stPlaBrk_mp : FromWorkspace  VariableName=testSig_APP_stPlaBrk_mp  Interpolate=off  OutputAfterFinalValue=Holding final value
  spec_Brk_st : FromWorkspace  VariableName=testSig_Brk_st  Interpolate=off  OutputAfterFinalValue=Holding final value
  spec_Brk_stMn : FromWorkspace  VariableName=testSig_Brk_stMn  Interpolate=off  OutputAfterFinalValue=Holding final value
  spec_Brk_stRed : FromWorkspace  VariableName=testSig_Brk_stRed  Interpolate=off  OutputAfterFinalValue=Holding final value
  spec_DSM_bAPPBrkDef : FromWorkspace  VariableName=testSig_DSM_bAPPBrkDef  Interpolate=off  OutputAfterFinalValue=Holding final value
  spec_DSM_bAPPVel : FromWorkspace  VariableName=testSig_DSM_bAPPVel  Interpolate=off  OutputAfterFinalValue=Holding final value
  spec_Epm_nEng : FromWorkspace  VariableName=testSig_Epm_nEng  Interpolate=off  OutputAfterFinalValue=Holding final value
  spec_VehV_v : FromWorkspace  VariableName=testSig_VehV_v  Interpolate=off  OutputAfterFinalValue=Holding final value
  testSignals : Outport
  wires:
  BC/1 -> testSignals/1
  spec_APP_rUnFlt/1 -> BC/1  "testSig_APP_rUnFlt"
  spec_APP_drUnFlt/1 -> BC/2  "testSig_APP_drUnFlt"
  spec_Brk_st/1 -> BC/3  "testSig_Brk_st"
  spec_Brk_stMn/1 -> BC/4  "testSig_Brk_stMn"
  spec_Brk_stRed/1 -> BC/5  "testSig_Brk_stRed"
  spec_DSM_bAPPBrkDef/1 -> BC/6  "testSig_DSM_bAPPBrkDef"
  spec_Epm_nEng/1 -> BC/7  "testSig_Epm_nEng"
  spec_VehV_v/1 -> BC/8  "testSig_VehV_v"
  spec_DSM_bAPPVel/1 -> BC/9  "testSig_DSM_bAPPVel"
  spec_APP_stPlaBrkDet_mp/1 -> BC/10  "testSig_APP_stPlaBrkDet_mp"
  spec_APP_stPlaBrkRst_mp/1 -> BC/11  "testSig_APP_stPlaBrkRst_mp"
  spec_APP_stPlaBrk_mp/1 -> BC/12  "testSig_APP_stPlaBrk_mp"

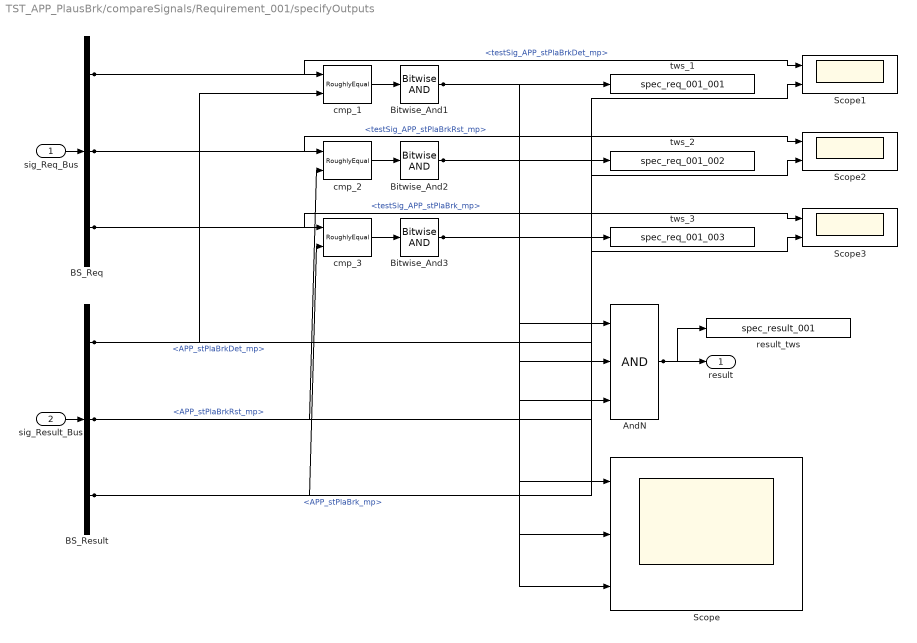
== system TST_APP_PlausBrk/compareSignals/Requirement_001/specifyOutputs ==
  sig_Req_Bus : Inport
  sig_Result_Bus : Inport  Port=2
  AndN : Logic  Inputs=3
  BS_Req : BusSelector  OutputSignals=testSig_APP_stPlaBrkDet_mp,testSig_APP_stPlaBrkRst_mp,testSig_APP_stPlaBrk_mp
  BS_Result : BusSelector  OutputSignals=APP_stPlaBrkDet_mp,APP_stPlaBrkRst_mp,APP_stPlaBrk_mp
  Bitwise_And1 : simulink/Logic and Bit Operations/Bitwise Operator  logicop=AND  UseBitMask=off  BitMask=bin2dec('11011001')  BitMaskRealWorld=Stored Integer
  Bitwise_And2 : simulink/Logic and Bit Operations/Bitwise Operator  logicop=AND  UseBitMask=off  BitMask=bin2dec('11011001')  BitMaskRealWorld=Stored Integer
  Bitwise_And3 : simulink/Logic and Bit Operations/Bitwise Operator  logicop=AND  UseBitMask=off  BitMask=bin2dec('11011001')  BitMaskRealWorld=Stored Integer
  Scope : Scope  NumInputPorts=3
  Scope1 : Scope  NumInputPorts=2
  Scope2 : Scope  NumInputPorts=2
  Scope3 : Scope  NumInputPorts=2
  cmp_1 : UnitTest_Lib/RoughlyEqual  slope=0.1
  cmp_2 : UnitTest_Lib/RoughlyEqual  slope=0.1
  cmp_3 : UnitTest_Lib/RoughlyEqual  slope=0.1
  result_tws : ToWorkspace  VariableName=spec_result_001
  tws_1 : ToWorkspace  VariableName=spec_req_001_001
  tws_2 : ToWorkspace  VariableName=spec_req_001_002
  tws_3 : ToWorkspace  VariableName=spec_req_001_003
  result : Outport
  wires:
  sig_Req_Bus/1 -> BS_Req/1
  sig_Result_Bus/1 -> BS_Result/1
  AndN/1 -> result/1, result_tws/1
  BS_Req/1 -> cmp_1/1, Scope1/1  "<testSig_APP_stPlaBrkDet_mp>"
  BS_Result/1 -> cmp_1/2, Scope1/2  "<APP_stPlaBrkDet_mp>"
  cmp_1/1 -> Bitwise_And1/1
  Bitwise_And1/1 -> tws_1/1, AndN/1, Scope/1
  BS_Req/2 -> cmp_2/1, Scope2/1  "<testSig_APP_stPlaBrkRst_mp>"
  BS_Result/2 -> cmp_2/2, Scope2/2  "<APP_stPlaBrkRst_mp>"
  cmp_2/1 -> Bitwise_And2/1
  Bitwise_And2/1 -> tws_2/1, AndN/2, Scope/2
  BS_Req/3 -> cmp_3/1, Scope3/1  "<testSig_APP_stPlaBrk_mp>"
  BS_Result/3 -> cmp_3/2, Scope3/2  "<APP_stPlaBrk_mp>"
  cmp_3/1 -> Bitwise_And3/1
  Bitwise_And3/1 -> tws_3/1, AndN/3, Scope/3

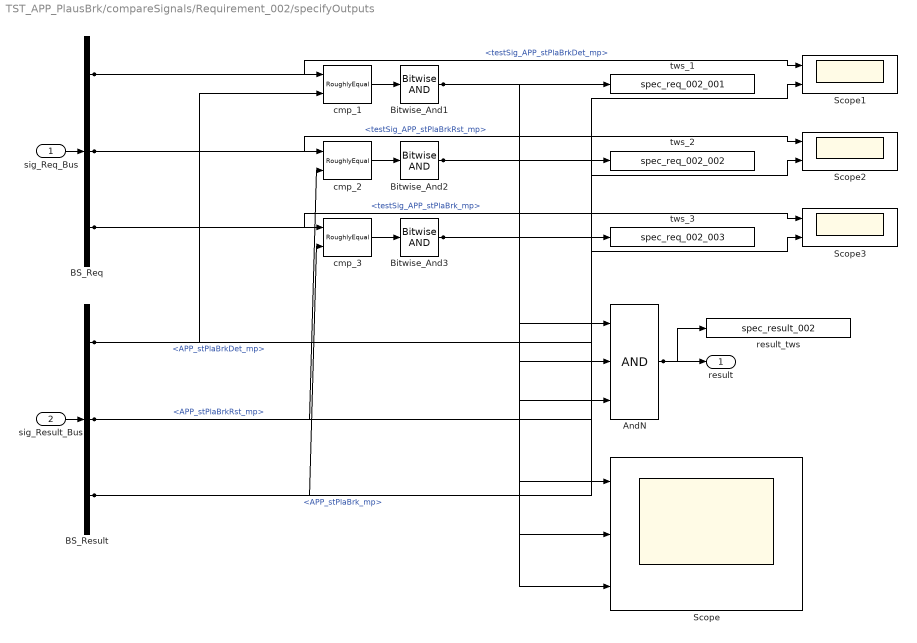
== system TST_APP_PlausBrk/compareSignals/Requirement_002/specifyOutputs ==
  sig_Req_Bus : Inport
  sig_Result_Bus : Inport  Port=2
  AndN : Logic  Inputs=3
  BS_Req : BusSelector  OutputSignals=testSig_APP_stPlaBrkDet_mp,testSig_APP_stPlaBrkRst_mp,testSig_APP_stPlaBrk_mp
  BS_Result : BusSelector  OutputSignals=APP_stPlaBrkDet_mp,APP_stPlaBrkRst_mp,APP_stPlaBrk_mp
  Bitwise_And1 : simulink/Logic and Bit Operations/Bitwise Operator  logicop=AND  UseBitMask=off  BitMask=bin2dec('11011001')  BitMaskRealWorld=Stored Integer
  Bitwise_And2 : simulink/Logic and Bit Operations/Bitwise Operator  logicop=AND  UseBitMask=off  BitMask=bin2dec('11011001')  BitMaskRealWorld=Stored Integer
  Bitwise_And3 : simulink/Logic and Bit Operations/Bitwise Operator  logicop=AND  UseBitMask=off  BitMask=bin2dec('11011001')  BitMaskRealWorld=Stored Integer
  Scope : Scope  NumInputPorts=3
  Scope1 : Scope  NumInputPorts=2
  Scope2 : Scope  NumInputPorts=2
  Scope3 : Scope  NumInputPorts=2
  cmp_1 : UnitTest_Lib/RoughlyEqual  slope=0.1
  cmp_2 : UnitTest_Lib/RoughlyEqual  slope=0.1
  cmp_3 : UnitTest_Lib/RoughlyEqual  slope=0.1
  result_tws : ToWorkspace  VariableName=spec_result_002
  tws_1 : ToWorkspace  VariableName=spec_req_002_001
  tws_2 : ToWorkspace  VariableName=spec_req_002_002
  tws_3 : ToWorkspace  VariableName=spec_req_002_003
  result : Outport
  wires:
  sig_Req_Bus/1 -> BS_Req/1
  sig_Result_Bus/1 -> BS_Result/1
  AndN/1 -> result/1, result_tws/1
  BS_Req/1 -> cmp_1/1, Scope1/1  "<testSig_APP_stPlaBrkDet_mp>"
  BS_Result/1 -> cmp_1/2, Scope1/2  "<APP_stPlaBrkDet_mp>"
  cmp_1/1 -> Bitwise_And1/1
  Bitwise_And1/1 -> tws_1/1, AndN/1, Scope/1
  BS_Req/2 -> cmp_2/1, Scope2/1  "<testSig_APP_stPlaBrkRst_mp>"
  BS_Result/2 -> cmp_2/2, Scope2/2  "<APP_stPlaBrkRst_mp>"
  cmp_2/1 -> Bitwise_And2/1
  Bitwise_And2/1 -> tws_2/1, AndN/2, Scope/2
  BS_Req/3 -> cmp_3/1, Scope3/1  "<testSig_APP_stPlaBrk_mp>"
  BS_Result/3 -> cmp_3/2, Scope3/2  "<APP_stPlaBrk_mp>"
  cmp_3/1 -> Bitwise_And3/1
  Bitwise_And3/1 -> tws_3/1, AndN/3, Scope/3

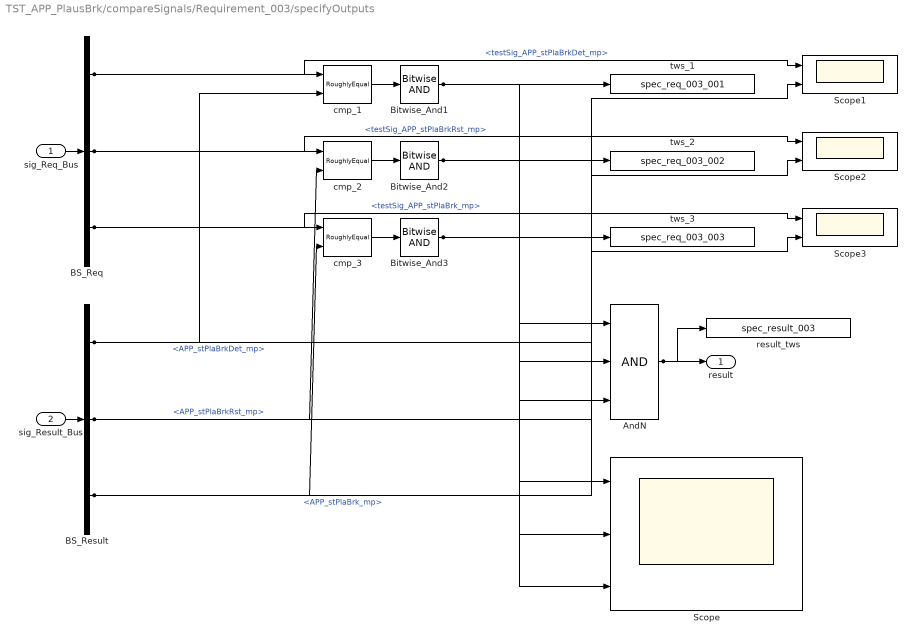
== system TST_APP_PlausBrk/compareSignals/Requirement_003/specifyOutputs ==
  sig_Req_Bus : Inport
  sig_Result_Bus : Inport  Port=2
  AndN : Logic  Inputs=3
  BS_Req : BusSelector  OutputSignals=testSig_APP_stPlaBrkDet_mp,testSig_APP_stPlaBrkRst_mp,testSig_APP_stPlaBrk_mp
  BS_Result : BusSelector  OutputSignals=APP_stPlaBrkDet_mp,APP_stPlaBrkRst_mp,APP_stPlaBrk_mp
  Bitwise_And1 : simulink/Logic and Bit Operations/Bitwise Operator  logicop=AND  UseBitMask=off  BitMask=bin2dec('11011001')  BitMaskRealWorld=Stored Integer
  Bitwise_And2 : simulink/Logic and Bit Operations/Bitwise Operator  logicop=AND  UseBitMask=off  BitMask=bin2dec('11011001')  BitMaskRealWorld=Stored Integer
  Bitwise_And3 : simulink/Logic and Bit Operations/Bitwise Operator  logicop=AND  UseBitMask=off  BitMask=bin2dec('11011001')  BitMaskRealWorld=Stored Integer
  Scope : Scope  NumInputPorts=3
  Scope1 : Scope  NumInputPorts=2
  Scope2 : Scope  NumInputPorts=2
  Scope3 : Scope  NumInputPorts=2
  cmp_1 : UnitTest_Lib/RoughlyEqual  slope=0.1
  cmp_2 : UnitTest_Lib/RoughlyEqual  slope=0.1
  cmp_3 : UnitTest_Lib/RoughlyEqual  slope=0.1
  result_tws : ToWorkspace  VariableName=spec_result_003
  tws_1 : ToWorkspace  VariableName=spec_req_003_001
  tws_2 : ToWorkspace  VariableName=spec_req_003_002
  tws_3 : ToWorkspace  VariableName=spec_req_003_003
  result : Outport
  wires:
  sig_Req_Bus/1 -> BS_Req/1
  sig_Result_Bus/1 -> BS_Result/1
  AndN/1 -> result/1, result_tws/1
  BS_Req/1 -> cmp_1/1, Scope1/1  "<testSig_APP_stPlaBrkDet_mp>"
  BS_Result/1 -> cmp_1/2, Scope1/2  "<APP_stPlaBrkDet_mp>"
  cmp_1/1 -> Bitwise_And1/1
  Bitwise_And1/1 -> tws_1/1, AndN/1, Scope/1
  BS_Req/2 -> cmp_2/1, Scope2/1  "<testSig_APP_stPlaBrkRst_mp>"
  BS_Result/2 -> cmp_2/2, Scope2/2  "<APP_stPlaBrkRst_mp>"
  cmp_2/1 -> Bitwise_And2/1
  Bitwise_And2/1 -> tws_2/1, AndN/2, Scope/2
  BS_Req/3 -> cmp_3/1, Scope3/1  "<testSig_APP_stPlaBrk_mp>"
  BS_Result/3 -> cmp_3/2, Scope3/2  "<APP_stPlaBrk_mp>"
  cmp_3/1 -> Bitwise_And3/1
  Bitwise_And3/1 -> tws_3/1, AndN/3, Scope/3

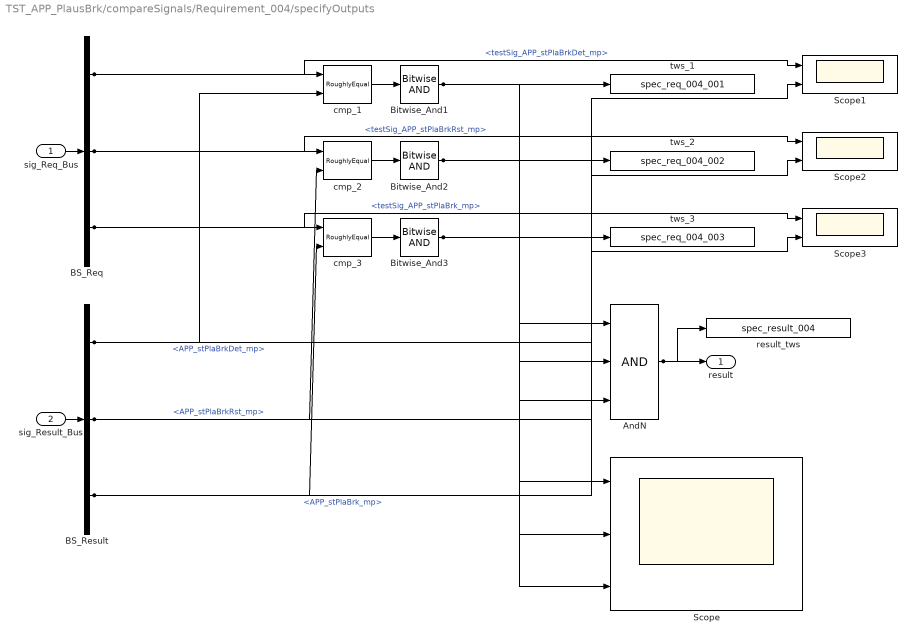
== system TST_APP_PlausBrk/compareSignals/Requirement_004/specifyOutputs ==
  sig_Req_Bus : Inport
  sig_Result_Bus : Inport  Port=2
  AndN : Logic  Inputs=3
  BS_Req : BusSelector  OutputSignals=testSig_APP_stPlaBrkDet_mp,testSig_APP_stPlaBrkRst_mp,testSig_APP_stPlaBrk_mp
  BS_Result : BusSelector  OutputSignals=APP_stPlaBrkDet_mp,APP_stPlaBrkRst_mp,APP_stPlaBrk_mp
  Bitwise_And1 : simulink/Logic and Bit Operations/Bitwise Operator  logicop=AND  UseBitMask=off  BitMask=bin2dec('11011001')  BitMaskRealWorld=Stored Integer
  Bitwise_And2 : simulink/Logic and Bit Operations/Bitwise Operator  logicop=AND  UseBitMask=off  BitMask=bin2dec('11011001')  BitMaskRealWorld=Stored Integer
  Bitwise_And3 : simulink/Logic and Bit Operations/Bitwise Operator  logicop=AND  UseBitMask=off  BitMask=bin2dec('11011001')  BitMaskRealWorld=Stored Integer
  Scope : Scope  NumInputPorts=3
  Scope1 : Scope  NumInputPorts=2
  Scope2 : Scope  NumInputPorts=2
  Scope3 : Scope  NumInputPorts=2
  cmp_1 : UnitTest_Lib/RoughlyEqual  slope=0.1
  cmp_2 : UnitTest_Lib/RoughlyEqual  slope=0.1
  cmp_3 : UnitTest_Lib/RoughlyEqual  slope=0.1
  result_tws : ToWorkspace  VariableName=spec_result_004
  tws_1 : ToWorkspace  VariableName=spec_req_004_001
  tws_2 : ToWorkspace  VariableName=spec_req_004_002
  tws_3 : ToWorkspace  VariableName=spec_req_004_003
  result : Outport
  wires:
  sig_Req_Bus/1 -> BS_Req/1
  sig_Result_Bus/1 -> BS_Result/1
  AndN/1 -> result/1, result_tws/1
  BS_Req/1 -> cmp_1/1, Scope1/1  "<testSig_APP_stPlaBrkDet_mp>"
  BS_Result/1 -> cmp_1/2, Scope1/2  "<APP_stPlaBrkDet_mp>"
  cmp_1/1 -> Bitwise_And1/1
  Bitwise_And1/1 -> tws_1/1, AndN/1, Scope/1
  BS_Req/2 -> cmp_2/1, Scope2/1  "<testSig_APP_stPlaBrkRst_mp>"
  BS_Result/2 -> cmp_2/2, Scope2/2  "<APP_stPlaBrkRst_mp>"
  cmp_2/1 -> Bitwise_And2/1
  Bitwise_And2/1 -> tws_2/1, AndN/2, Scope/2
  BS_Req/3 -> cmp_3/1, Scope3/1  "<testSig_APP_stPlaBrk_mp>"
  BS_Result/3 -> cmp_3/2, Scope3/2  "<APP_stPlaBrk_mp>"
  cmp_3/1 -> Bitwise_And3/1
  Bitwise_And3/1 -> tws_3/1, AndN/3, Scope/3
